simulink model "test"  (R2017a)
settings: Solver=VariableStepAuto  StartTime=0.0  StopTime=Tf  MaxStep=1e-6  RelTol=1e-3
values from neighbouring files (symbols this model uses):
  K = 0.01    [HW2_driver.m]    (also in HW3_driver.m = 4; Lab_6.m = 1.5; Lab_7.m = 1.5; test_driver.m = 3)
  tau = 0.000375    [HW2_driver.m]    (also in HW3_driver.m = 6.67; Lab_6.m = 0.001; Lab_7.m = 0.001; test_driver.m = 0.2)
  y0 = 0    [HW2_driver.m]    (also in HW3_driver.m; test_driver.m)
settings Model: Creator=localmgr  LastModifiedBy=localmgr

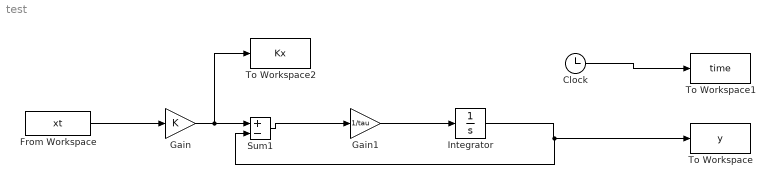
== system test ==
  Clock : Clock
  From Workspace : FromWorkspace  VariableName=xt  SampleTime=0
  Gain : Gain  Gain=K
  Gain1 : Gain  Gain=1/tau
  Integrator : Integrator  InitialCondition=y0
  Sum1 : Sum  Inputs=|+|-|
  To Workspace : ToWorkspace  VariableName=y  SampleTime=-1
  To Workspace1 : ToWorkspace  VariableName=time  SampleTime=-1
  To Workspace2 : ToWorkspace  VariableName=Kx  SampleTime=-1
  wires:
  Gain/1 -> To Workspace2/1, Sum1/1
  Sum1/1 -> Gain1/1
  Gain1/1 -> Integrator/1
  Integrator/1 -> To Workspace/1, Sum1/2
  Clock/1 -> To Workspace1/1
  From Workspace/1 -> Gain/1
